simulink model "Plant"  (R2020a)
settings: Solver=VariableStepAuto  StartTime=0.0  StopTime=10.0  RelTol=1e-3
undefined symbols (not defined in the file): b, J, K, L, R
settings Model: Creator=sreeram  LastModifiedBy=sreeram
settings DataIOCC: SaveOutput=off  SaveTime=off

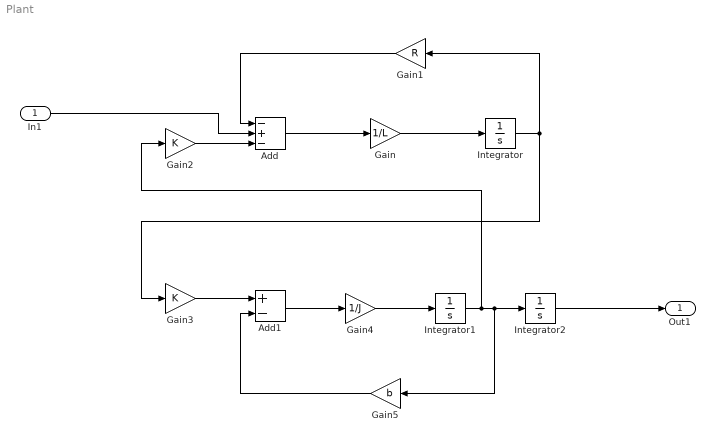
== system Plant ==
  In1 : Inport  OutDataTypeStr=double  PortDimensions=1  SampleTime=0
  Add : Sum  Inputs=-+-
  Add1 : Sum  Inputs=+-
  Gain : Gain  Gain=1/L
  Gain1 : Gain  Gain=R
  Gain2 : Gain  Gain=K
  Gain3 : Gain  Gain=K
  Gain4 : Gain  Gain=1/J
  Gain5 : Gain  Gain=b
  Integrator : Integrator
  Integrator1 : Integrator
  Integrator2 : Integrator
  Out1 : Outport  OutDataTypeStr=double  PortDimensions=1  SampleTime=0
  wires:
  Gain4/1 -> Integrator1/1
  Add/1 -> Gain/1
  Add1/1 -> Gain4/1
  Gain1/1 -> Add/1
  Gain/1 -> Integrator/1
  Gain3/1 -> Add1/1
  Integrator/1 -> Gain1/1, Gain3/1
  Gain5/1 -> Add1/2
  Gain2/1 -> Add/3
  Integrator1/1 -> Integrator2/1, Gain5/1, Gain2/1
  Integrator2/1 -> Out1/1
  In1/1 -> Add/2
